simulink library "lib_Driver"  (R2017b)
settings: Solver=VariableStepAuto  StartTime=0.0  StopTime=10.0  RelTol=1e-3
undefined symbols (not defined in the file): ABSEnable, cal, CS_On_Control, KeyPosition, mph2ms, RegenBrkDisable, ShiftLeverPosition, Speed, SW_CS_ON, SW_Engine_ON, time
libraries: simulink x5, Utility x1
settings Model: Creator=Di Russo  LastModifiedBy=Lyu19
settings CodeAppCC: StateflowObjectComments=on

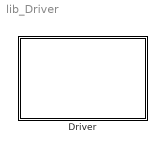
== system lib_Driver ==
  Driver : Subsystem
      mask Display: image('Images/Driver.jpg')

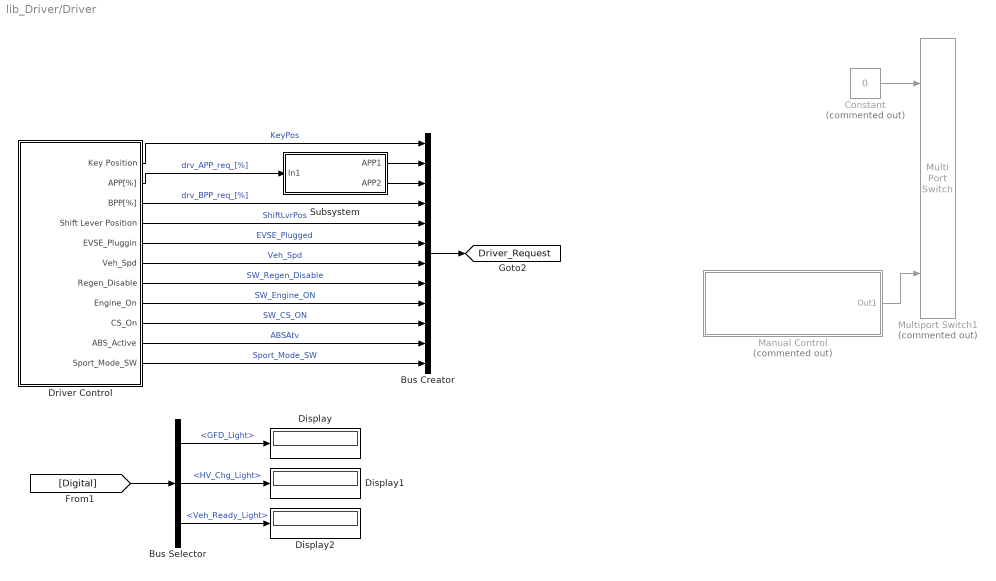
== system lib_Driver/Driver ==
  Bus Creator : BusCreator  Inputs=12
  Bus Selector : BusSelector  OutputSignals=GFD_Light,HV_Chg_Light,Veh_Ready_Light
  Constant : Constant  Commented=on  Value=0
  Display : Display
  Display1 : Display
  Display2 : Display
  Driver Control : Subsystem
  Manual Control : Subsystem  Commented=on
  Multiport Switch1 : MultiPortSwitch  Commented=on  DataPortOrder=Zero-based contiguous  Inputs=2
  Subsystem : Subsystem
  tag scope: Driver_Request=global
  wires:
  Driver Control/1(Key Position) -> Bus Creator/1  "KeyPos"
  Driver Control/2(APP[%]) -> Subsystem/1(In1)  "drv_APP_req_[%]"
  Driver Control/3(BPP[%]) -> Bus Creator/4  "drv_BPP_req_[%]"
  Driver Control/4(Shift Lever Position) -> Bus Creator/5  "ShiftLvrPos"
  Driver Control/5(EVSE_Pluggin) -> Bus Creator/6  "EVSE_Plugged"
  Constant/1 -> Multiport Switch1/1
  Manual Control/1(Out1) -> Multiport Switch1/3
  Bus Creator/1 -> [Driver_Request]
  Driver Control/6(Veh_Spd) -> Bus Creator/7  "Veh_Spd"
  Driver Control/7(Regen_Disable) -> Bus Creator/8  "SW_Regen_Disable"
  Driver Control/8(Engine_On) -> Bus Creator/9  "SW_Engine_ON"
  Driver Control/9(CS_On) -> Bus Creator/10  "SW_CS_ON"
  [Digital] -> Bus Selector/1
  Bus Selector/1 -> Display/1  "<GFD_Light>"
  Bus Selector/2 -> Display1/1  "<HV_Chg_Light>"
  Bus Selector/3 -> Display2/1  "<Veh_Ready_Light>"
  Subsystem/1(APP1) -> Bus Creator/2
  Subsystem/2(APP2) -> Bus Creator/3
  Driver Control/10(ABS_Active) -> Bus Creator/11  "ABSAtv"
  Driver Control/11(Sport_Mode_SW) -> Bus Creator/12  "Sport_Mode_SW"

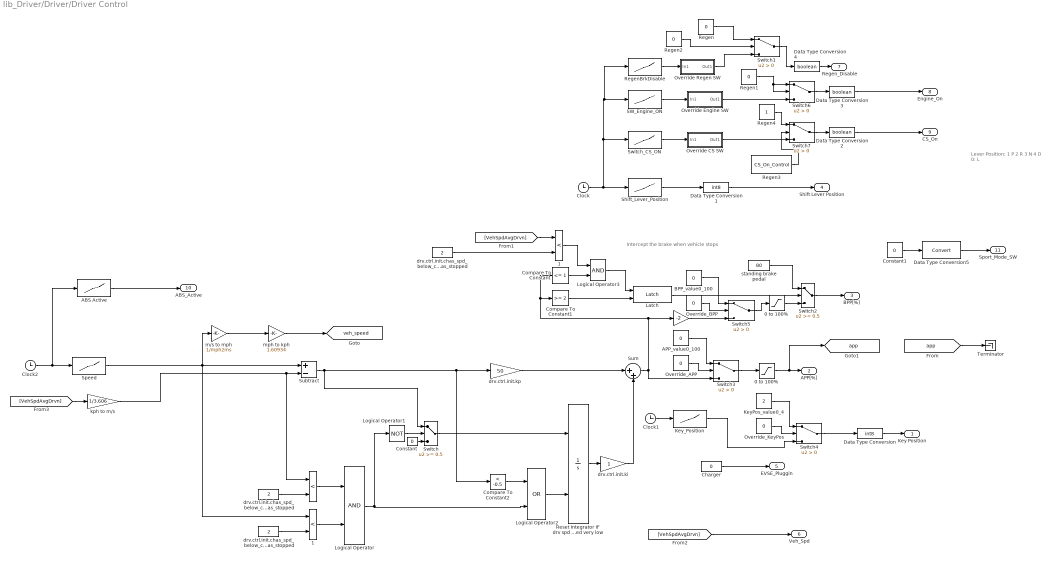
== system lib_Driver/Driver/Driver Control ==
  note: Lever Position:
      | 1 P
      | 2 R
      | 3 N
      | 4 D
      | 0: L
  note: Intercept the brake when vehicle stops
  " " : Gain  Gain=-2
  "    " : RelationalOperator  Operator=<  RndMeth=Nearest  InputSameDT=on
  "    1" : RelationalOperator  Operator=<  RndMeth=Nearest  InputSameDT=on
  "  1" : RelationalOperator  Operator=<  RndMeth=Nearest  InputSameDT=on
  0 to 100% : Saturate  UpperLimit=100  LowerLimit=0
  "0 to 100% " : Saturate  UpperLimit=100  LowerLimit=0
  ABS Active : Lookup  InputValues=time  Table=ABSEnable
  APP_value0_100 : Constant  Value=0
  BPP_value0_100 : Constant  Value=0
  Charger : Constant  Value=0
  Clock : Clock
  Clock1 : Clock
  Clock2 : Clock
  Compare To Constant : simulink/Logic and Bit Operations/Compare To Constant  relop=<=  const=1  OutDataTypeStr=boolean
  Compare To Constant1 : simulink/Logic and Bit Operations/Compare To Constant  relop=>=  const=2  OutDataTypeStr=boolean
  Compare To Constant2 : simulink/Logic and Bit Operations/Compare To Constant  relop=<  const=-0.5  OutDataTypeStr=boolean
  Constant : Constant  Value=0
  Constant1 : Constant  Value=0
  Data Type Conversion : DataTypeConversion  OutDataTypeStr=int8
  Data Type Conversion1 : DataTypeConversion  OutDataTypeStr=int8
  Data Type Conversion2 : DataTypeConversion  OutDataTypeStr=boolean
  Data Type Conversion3 : DataTypeConversion  OutDataTypeStr=boolean
  Data Type Conversion4 : DataTypeConversion  OutDataTypeStr=boolean
  Data Type Conversion5 : DataTypeConversion
  KeyPos_value0_4 : Constant  Value=2
  Key_Position : Lookup  InputValues=time  Table=KeyPosition
  Latch : Utility/Latch
  Logical Operator : Logic  AllPortsSameDT=off  OutDataTypeStr=boolean
  Logical Operator1 : Logic  Operator=NOT  AllPortsSameDT=off  OutDataTypeStr=boolean
  Logical Operator2 : Logic  Operator=OR  AllPortsSameDT=off  OutDataTypeStr=boolean
  Logical Operator3 : Logic  AllPortsSameDT=off  OutDataTypeStr=boolean
  Override CS SW : Subsystem
  Override Engine SW : Subsystem
  Override Regen SW : Subsystem
  Override_APP : Constant  Value=0
  Override_BPP : Constant  Value=0
  Override_KeyPos : Constant  Value=0
  Regen : Constant  Value=0
  Regen1 : Constant  Value=0
  Regen2 : Constant  Value=0
  Regen3 : Constant  Value=CS_On_Control
  Regen4 : Constant
  RegenBrkDisable : Lookup  InputValues=time  Table=RegenBrkDisable
  Reset Integrator IF drv spd dmd very low AND AND current vehicle speed very low : Integrator  ExternalReset=either
  SW_Engine_ON : Lookup  InputValues=time  Table=SW_Engine_ON
  Shift_Lever_Position : Lookup  InputValues=time  Table=ShiftLeverPosition
  Speed : Lookup  InputValues=time  Table=Speed
  Subtract : Sum  Inputs=+-
  Sum : Sum  Inputs=|++  SaturateOnIntegerOverflow=on  InputSameDT=on  OutDataTypeStr=Inherit: Same as first input
  Switch : Switch  Threshold=0.5
  Switch{1,3..7} (6 alike) : Switch  Criteria=u2 > Threshold
  Switch2 : Switch  Threshold=0.5
  Switch_CS_ON : Lookup  InputValues=time  Table=SW_CS_ON
  Terminator : Terminator
  "drv.ctrl.init.chas_spd_below_chas_stopped " : Constant  Value=2
  "drv.ctrl.init.chas_spd_below_chas_stopped " : Constant  Value=2
  "drv.ctrl.init.chas_spd_below_chas_stopped " : Constant  Value=2
  drv.ctrl.init.ki : Gain  SaturateOnIntegerOverflow=on  OutDataTypeStr=Inherit: Same as input  ParamDataTypeStr=Inherit: Same as input
  drv.ctrl.init.kp : Gain  Gain=50  SaturateOnIntegerOverflow=on  OutDataTypeStr=Inherit: Same as input  ParamDataTypeStr=Inherit: Same as input
  kph to m/s : Gain  Gain=1/3.606  SaturateOnIntegerOverflow=on  OutDataTypeStr=Inherit: Same as input  ParamDataTypeStr=Inherit: Same as input
  m/s to mph : Gain  Gain=1/mph2ms
  mph to kph : Gain  Gain=1.60934
  standing brake pedal : Constant  Value=80
  Key Position : Outport
  APP[%] : Outport  Port=2
  BPP[%] : Outport  Port=3
  Shift Lever Position : Outport  Port=4
  EVSE_Pluggin : Outport  Port=5
  Veh_Spd : Outport  Port=6
  Regen_Disable : Outport  Port=7
  Engine_On : Outport  Port=8
  CS_On : Outport  Port=9
  ABS_Active : Outport  Port=10
  Sport_Mode_SW : Outport  Port=11
  tag scope: app=global, veh_speed=global
  wires:
  drv.ctrl.init.kp/1 -> Sum/1
  "    "/1 -> Logical Operator/1
  Constant/1 -> Switch/3
  Reset Integrator IF drv spd dmd very low AND AND current vehicle speed very low/1 -> drv.ctrl.init.ki/1
  Logical Operator1/1 -> Switch/2
  "drv.ctrl.init.chas_spd_below_chas_stopped "/1 -> "    "/2
  Switch/1 -> Reset Integrator IF drv spd dmd very low AND AND current vehicle speed very low/1
  Logical Operator2/1 -> Reset Integrator IF drv spd dmd very low AND AND current vehicle speed very low/2
  "drv.ctrl.init.chas_spd_below_chas_stopped "/1 -> "  1"/2
  drv.ctrl.init.ki/1 -> Sum/2
  "  1"/1 -> Logical Operator/2
  Logical Operator/1 -> Logical Operator2/2, Logical Operator1/1
  "0 to 100% "/1 -> Switch2/3
  " "/1 -> Switch5/3
  [VehSpdAvgDrvn] -> kph to m/s/1
  standing brake pedal/1 -> Switch2/1
  Switch2/1 -> BPP[%]/1
  [VehSpdAvgDrvn] -> "    1"/1
  "drv.ctrl.init.chas_spd_below_chas_stopped "/1 -> "    1"/2
  "    1"/1 -> Logical Operator3/1
  Sum/1 -> Compare To Constant1/1, Compare To Constant/1, " "/1, Switch3/3
  Logical Operator3/1 -> Latch/1
  Compare To Constant/1 -> Logical Operator3/2
  Compare To Constant1/1 -> Latch/2
  Data Type Conversion/1 -> Key Position/1
  Data Type Conversion1/1 -> Shift Lever Position/1
  Charger/1 -> EVSE_Pluggin/1
  Subtract/1 -> Compare To Constant2/1, drv.ctrl.init.kp/1, Switch/1
  Compare To Constant2/1 -> Logical Operator2/1
  Clock/1 -> RegenBrkDisable/1, SW_Engine_ON/1, Switch_CS_ON/1, Shift_Lever_Position/1
  Clock1/1 -> Key_Position/1
  Clock2/1 -> ABS Active/1, Speed/1
  m/s to mph/1 -> mph to kph/1
  mph to kph/1 -> [veh_speed]
  0 to 100%/1 -> [app], APP[%]/1
  Switch_CS_ON/1 -> Override CS SW/1(In1)
  SW_Engine_ON/1 -> Override Engine SW/1(In1)
  RegenBrkDisable/1 -> Override Regen SW/1(In1)
  Override Regen SW/1(Out1) -> Switch1/3
  Data Type Conversion2/1 -> CS_On/1
  Data Type Conversion4/1 -> Regen_Disable/1
  [VehSpdAvgDrvn] -> Veh_Spd/1
  Switch3/1 -> 0 to 100%/1
  Override_APP/1 -> Switch3/2
  APP_value0_100/1 -> Switch3/1
  Key_Position/1 -> Switch4/3
  Override_KeyPos/1 -> Switch4/2
  KeyPos_value0_4/1 -> Switch4/1
  Switch4/1 -> Data Type Conversion/1
  Latch/1 -> Switch2/2
  Override_BPP/1 -> Switch5/2
  BPP_value0_100/1 -> Switch5/1
  Switch5/1 -> "0 to 100% "/1
  Shift_Lever_Position/1 -> Data Type Conversion1/1
  Regen/1 -> Switch1/1
  Switch1/1 -> Data Type Conversion4/1
  Regen1/1 -> Switch6/2, Switch6/1
  Data Type Conversion3/1 -> Engine_On/1
  Override Engine SW/1(Out1) -> Switch6/3
  Switch6/1 -> Data Type Conversion3/1
  kph to m/s/1 -> Subtract/2, "    "/1
  ABS Active/1 -> ABS_Active/1
  Data Type Conversion5/1 -> Sport_Mode_SW/1
  Constant1/1 -> Data Type Conversion5/1
  Regen2/1 -> Switch1/2
  Switch7/1 -> Data Type Conversion2/1
  Override CS SW/1(Out1) -> Switch7/3
  Regen3/1 -> Switch7/2
  Regen4/1 -> Switch7/1
  [app] -> Terminator/1
  Speed/1 -> Subtract/1, m/s to mph/1, "  1"/1

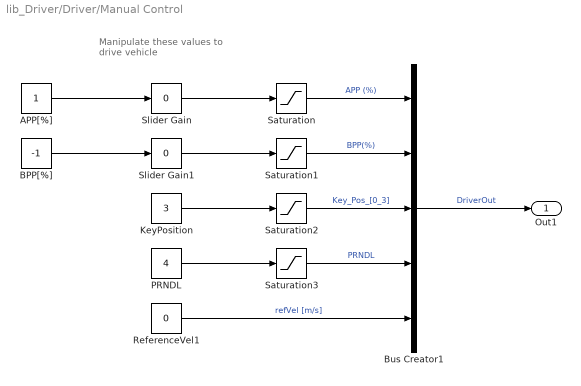
== system lib_Driver/Driver/Manual Control ==
  note: Manipulate these values
      | to drive vehicle
  APP[%] : Constant
  BPP[%] : Constant  Value=-1
  Bus Creator1 : BusCreator  Inputs=5
  KeyPosition : Constant  Value=3
  PRNDL : Constant  Value=4
  ReferenceVel1 : Constant  Value=0
  Saturation : Saturate  UpperLimit=100  LowerLimit=0
  Saturation1 : Saturate  UpperLimit=0  LowerLimit=-100
  Saturation2 : Saturate  UpperLimit=3  LowerLimit=0
  Saturation3 : Saturate  UpperLimit=4  LowerLimit=0
  Slider Gain : simulink/Math Operations/Slider Gain  gain=0  low=0  high=100
  Slider Gain1 : simulink/Math Operations/Slider Gain  gain=0  low=0  high=100
  Out1 : Outport
  wires:
  Saturation2/1 -> Bus Creator1/3  "Key_Pos_[0_3]"
  Saturation1/1 -> Bus Creator1/2  "BPP(%)"
  Saturation/1 -> Bus Creator1/1  "APP (%)"
  KeyPosition/1 -> Saturation2/1
  Bus Creator1/1 -> Out1/1  "DriverOut"
  BPP[%]/1 -> Slider Gain1/1
  APP[%]/1 -> Slider Gain/1
  ReferenceVel1/1 -> Bus Creator1/5  "refVel [m/s]"
  PRNDL/1 -> Saturation3/1
  Saturation3/1 -> Bus Creator1/4  "PRNDL"
  Slider Gain/1 -> Saturation/1
  Slider Gain1/1 -> Saturation1/1

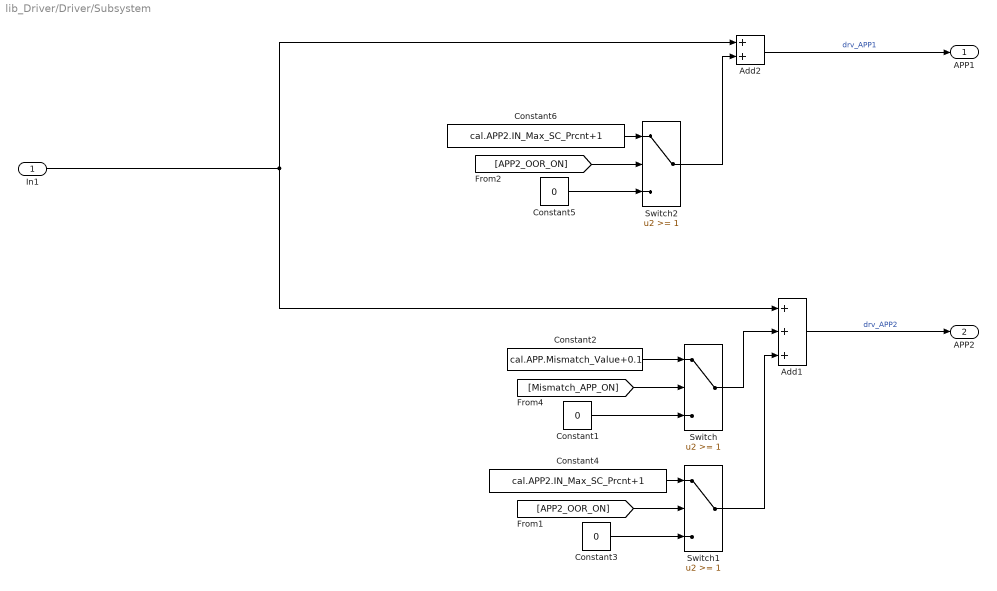
== system lib_Driver/Driver/Subsystem ==
  In1 : Inport
  Add1 : Sum  Inputs=+++
  Add2 : Sum
  Constant1 : Constant  Value=0
  Constant2 : Constant  Value=cal.APP.Mismatch_Value+0.1
  Constant3 : Constant  Value=0
  Constant4 : Constant  Value=cal.APP2.IN_Max_SC_Prcnt+1
  Constant5 : Constant  Value=0
  Constant6 : Constant  Value=cal.APP2.IN_Max_SC_Prcnt+1
  Switch : Switch  Threshold=1
  Switch1 : Switch  Threshold=1
  Switch2 : Switch  Threshold=1
  APP1 : Outport
  APP2 : Outport  Port=2
  wires:
  [Mismatch_APP_ON] -> Switch/2
  Switch/1 -> Add1/2
  Constant1/1 -> Switch/3
  Constant2/1 -> Switch/1
  Constant3/1 -> Switch1/3
  Constant4/1 -> Switch1/1
  [APP2_OOR_ON] -> Switch1/2
  Switch1/1 -> Add1/3
  Add1/1 -> APP2/1  "drv_APP2"
  In1/1 -> Add2/1, Add1/1
  Constant5/1 -> Switch2/3
  Constant6/1 -> Switch2/1
  [APP2_OOR_ON] -> Switch2/2
  Add2/1 -> APP1/1  "drv_APP1"
  Switch2/1 -> Add2/2

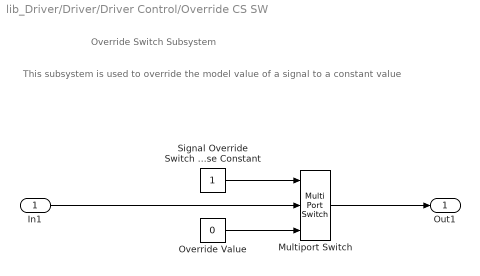
== system lib_Driver/Driver/Driver Control/Override CS SW ==
  note: Override Switch Subsystem
  note: This subsystem is used to override the model value of a signal to a constant value
  In1 : Inport
  Multiport Switch : MultiPortSwitch  DataPortOrder=Zero-based contiguous  Inputs=2  zeroidx=on
  Override Value : Constant  Value=0  OutDataTypeStr=double
  Signal Override Switch 0 = Use Model 1 = Use Constant : Constant
  Out1 : Outport
  wires:
  Override Value/1 -> Multiport Switch/3
  Multiport Switch/1 -> Out1/1
  In1/1 -> Multiport Switch/2
  Signal Override Switch 0 = Use Model 1 = Use Constant/1 -> Multiport Switch/1

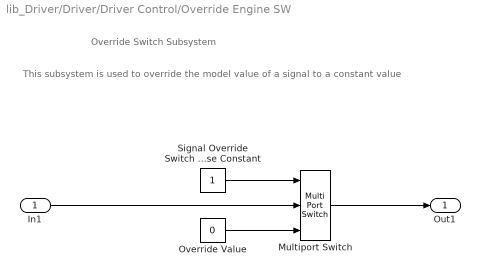
== system lib_Driver/Driver/Driver Control/Override Engine SW ==
  note: This subsystem is used to override the model value of a signal to a constant value
  note: Override Switch Subsystem
  In1 : Inport
  Multiport Switch : MultiPortSwitch  DataPortOrder=Zero-based contiguous  Inputs=2  zeroidx=on
  Override Value : Constant  Value=0  OutDataTypeStr=double
  Signal Override Switch 0 = Use Model 1 = Use Constant : Constant
  Out1 : Outport
  wires:
  Signal Override Switch 0 = Use Model 1 = Use Constant/1 -> Multiport Switch/1
  In1/1 -> Multiport Switch/2
  Multiport Switch/1 -> Out1/1
  Override Value/1 -> Multiport Switch/3

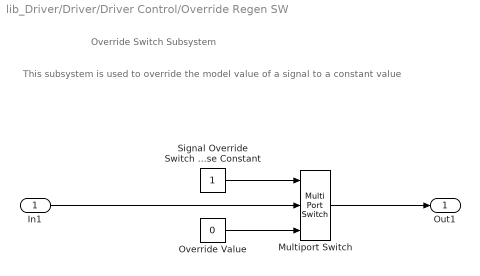
== system lib_Driver/Driver/Driver Control/Override Regen SW ==
  note: Override Switch Subsystem
  note: This subsystem is used to override the model value of a signal to a constant value
  In1 : Inport
  Multiport Switch : MultiPortSwitch  DataPortOrder=Zero-based contiguous  Inputs=2  zeroidx=on
  Override Value : Constant  Value=0  OutDataTypeStr=double
  Signal Override Switch 0 = Use Model 1 = Use Constant : Constant
  Out1 : Outport
  wires:
  Override Value/1 -> Multiport Switch/3
  Multiport Switch/1 -> Out1/1
  In1/1 -> Multiport Switch/2
  Signal Override Switch 0 = Use Model 1 = Use Constant/1 -> Multiport Switch/1
